simulink model "ParentsPhone_fuzzyLogic"  (R2024a)
settings: Solver=FixedStepAuto  StartTime=0.0  StopTime=inf  RelTol=1e-3
undefined symbols (not defined in the file): Altitude, Child, Latitude, Longitude, ParentsPhome, Voice
libraries: androidcommunicationlib x4, androiduilib x4, androidaudiovideolib x1
settings Model: Creator=Omkar R Prabhu  LastModifiedBy=Omkar R Prabhu
settings OptimizationCC: EnhancedBackFolding=on  PassReuseOutputArgsAs=Individual arguments  ZeroExternalMemoryAtStartup=off  ZeroInternalMemoryAtStartup=off  MaxStackSize=64  OptimizeBlockOrder=speed  DifferentSizesBufferReuse=on  OptimizationCustomize=off  EfficientTunableParamExpr=on
settings DebuggingCC: ParameterTunabilityLossMsg=error
settings HardwareCC: ProdBitPerPointer=32  ProdBitPerSizeT=32  ProdBitPerPtrDiffT=32  ProdLargestAtomicInteger=Long  ProdLargestAtomicFloat=Double  ProdWordSize=32  ProdHWDeviceType=ARM Compatible->ARM Cortex  UseEmbeddedCoderFeatures=off  UseSimulinkCoderFeatures=off
settings SFSimCC: MATLABDynamicMemAlloc=off
settings RTWCC: Description=Embedded Coder  SystemTargetFile=ert.tlc  HardwareBoard=Android Device  TLCOptions="-aInlineSetEventsForThisBaseRateFcn=TLC_FALSE -aSuppressMultiTaskScheduler=TLC_FALSE  -aRateBasedStepFcn=0"  TemplateMakefile=ert_default_tmf  RTWVerbose=off  Toolchain=Android SDK/NDK Tools
settings CodeAppCC: ForceParamTrailComments=on  IgnoreCustomStorageClasses=off  OperatorAnnotations=on  SimulinkDataObjDesc=on  SFDataObjDesc=on  InsertBlockDesc=on
settings ERTTargetCC: SupportNonInlinedSFcns=on

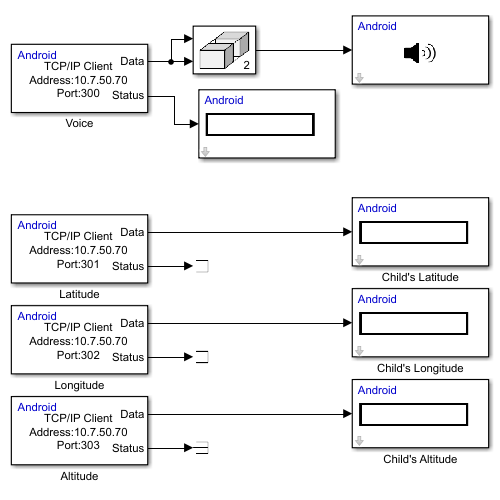
[thumbnail: Simulink's stored preview of the top-level diagram]
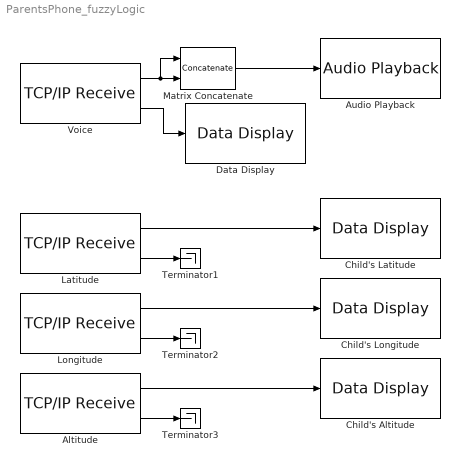
== system ParentsPhone_fuzzyLogic ==
  Altitude : androidcommunicationlib/TCP//IP Receive  TCPReceiveId=ParentsPhome/Altitude  Mode_=Client  LocalServerPort_=25000  RemoteAddr_=10.7.50.70  RemoteServerPort_=303  DataType_=uint8  DataSize_=1  SampleTime_=0.1  ClientPortBindingSelection_=off  ClientPortToBind_=35000  BlockingMode_=off  BlockTimeout_=0.1
  Audio Playback : androidaudiovideolib/Audio Playback  SampleFreq=44100  AudioSamplingFreq=44100  SampleTime=0.1  DeviceStr=0  QueueDuration=0  BlockPlatform=Android
  Child's Altitude : androiduilib/Data Display  DataDisplayId=ParentsPhome/Child's_Altitude  Format=Float  Precision=6  SimulateUsing=Code generation  blockPlatform=Android
  Child's Latitude : androiduilib/Data Display  DataDisplayId=ParentsPhome/Child's_Latitude  Format=Float  Precision=6  SimulateUsing=Code generation  blockPlatform=Android
  Child's Longitude : androiduilib/Data Display  DataDisplayId=ParentsPhome/Child's_Longitude  Format=Float  Precision=6  SimulateUsing=Code generation  blockPlatform=Android
  Data Display : androiduilib/Data Display  Format=Float  Precision=6  SimulateUsing=Code generation  blockPlatform=Android
  Latitude : androidcommunicationlib/TCP//IP Receive  TCPReceiveId=ParentsPhome/Latitude  Mode_=Client  LocalServerPort_=25000  RemoteAddr_=10.7.50.70  RemoteServerPort_=301  DataType_=uint8  DataSize_=1  SampleTime_=0.1  ClientPortBindingSelection_=off  ClientPortToBind_=35000  BlockingMode_=off  BlockTimeout_=0.1
  Longitude : androidcommunicationlib/TCP//IP Receive  TCPReceiveId=ParentsPhome/Longitude  Mode_=Client  LocalServerPort_=25000  RemoteAddr_=10.7.50.70  RemoteServerPort_=302  DataType_=uint8  DataSize_=1  SampleTime_=0.1  ClientPortBindingSelection_=off  ClientPortToBind_=35000  BlockingMode_=off  BlockTimeout_=0.1
  Matrix Concatenate : Concatenate  Mode=Multidimensional array  ConcatenateDimension=2
  Terminator1 : Terminator
  Terminator2 : Terminator
  Terminator3 : Terminator
  Voice : androidcommunicationlib/TCP//IP Receive  TCPReceiveId=ParentsPhome/Voice  Mode_=Client  LocalServerPort_=25000  RemoteAddr_=10.7.50.70  RemoteServerPort_=300  DataType_=int16  DataSize_=4410  SampleTime_=0.1  ClientPortBindingSelection_=off  ClientPortToBind_=35000  BlockingMode_=off  BlockTimeout_=0.1
  wires:
  Latitude/1 -> Child's Latitude/1
  Altitude/2 -> Terminator3/1
  Longitude/2 -> Terminator2/1
  Longitude/1 -> Child's Longitude/1
  Latitude/2 -> Terminator1/1
  Altitude/1 -> Child's Altitude/1
  Voice/1 -> Matrix Concatenate/1, Matrix Concatenate/2
  Matrix Concatenate/1 -> Audio Playback/1
  Voice/2 -> Data Display/1
